simulink model "LdAfsDblSlave_Runner"  (R2020b)
settings: configuration reference "VLS_Standard_Configuration" (kept outside this file)
settings Model: DataDictionary=LdAfsDblSlaveDD.sldd  Creator=ahashem  LastModifiedBy=ahashem
settings ConfigSetRef: SourceName=VLS_Standard_Configuration

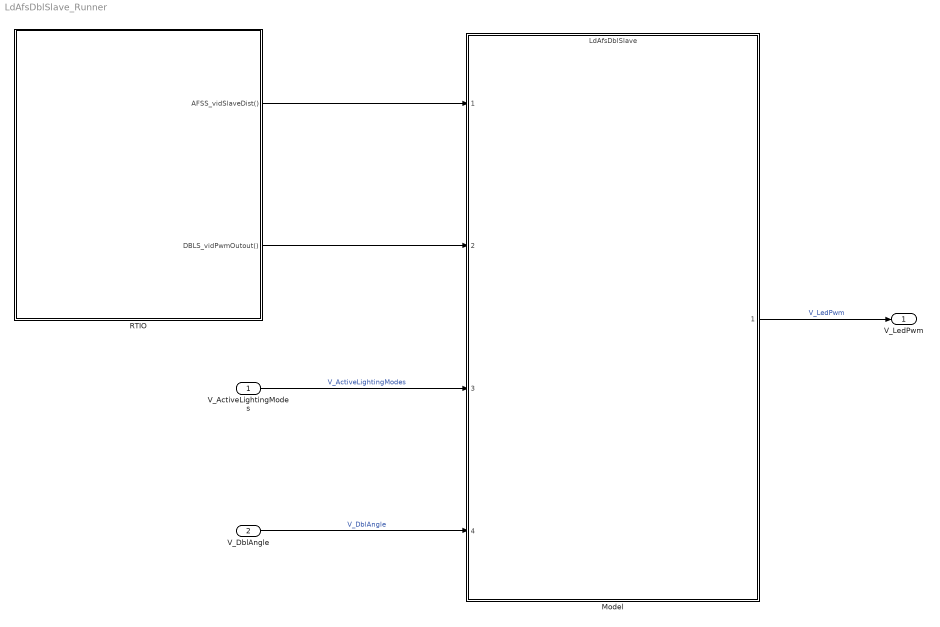
== system LdAfsDblSlave_Runner ==
  V_ActiveLightingModes : Inport
  V_DblAngle : Inport  Port=2
  Model : ModelReference  ModelNameDialog=LdAfsDblSlave.slx  SimulationMode=Normal  ScheduleRates=on  ModelReferenceVersion=1.29
  RTIO : Stateflow chart  TreatAsAtomicUnit=on  SystemSampleTime=0.02
  V_LedPwm : Outport  VectorParamsAs1DForOutWhenUnconnected=off
  wires:
  RTIO/1(AFSS_vidSlaveDist()) -> Model/1
  RTIO/2(DBLS_vidPwmOutout()) -> Model/2
  V_ActiveLightingModes/1 -> Model/3  "V_ActiveLightingModes"
  V_DblAngle/1 -> Model/4  "V_DblAngle"
  Model/1 -> V_LedPwm/1  "V_LedPwm"

== stateflow chart LdAfsDblSlave_Runner/RTIO ==
  state Schedule
    on every(1,tick):
    send(AFSS_vidSlaveDist);
    send(DBLS_vidPwmOutout);
  (default) -> Schedule
  events: AFSS_vidSlaveDist output FUNCTION_CALL_EVENT; DBLS_vidPwmOutout output FUNCTION_CALL_EVENT
